simulink model "Drone_BBall_Developer"  (R2020a)
settings: Solver=FixedStepAuto  StartTime=0.0  StopTime=60  FixedStep=.001  RelTol=1e-3
values from neighbouring files (symbols this model uses):
  b = .25*m    (= 0.25)    [Run_Match.m]
  b_ball = .02*m_ball    (= 0.01)    [Run_Match.m]
  b_F_hook = 100    [Run_Match.m]
  b_F_hoop = m_ball * 50    (= 25)    [Run_Match.m]
  b_F_R = m * 20    (= 20)    [Run_Match.m]
  b_F_R_ball = m_ball * 10    (= 5)    [Run_Match.m]
  b_F_R_hook = m_hook * 100    (= 10)    [Run_Match.m]
  B_hook = r_hook^2*6*m_ball*g    (= 0.2943)    [Run_Match.m]
  b_hook = 0.05*m_hook    (= 0.005)    [Run_Match.m]
  b_tether = 1    [Run_Match.m]
  b_th = .1*J    (= 0.0192708333333)    [Run_Match.m]
  b_th_ball = .05*J_ball    (= 0.0009)    [Run_Match.m]
  b_x_net = 80*m_ball*g    (= 392.4)    [Run_Match.m]
  b_y_net = .4*m_ball*g    (= 1.962)    [Run_Match.m]
  drone = struct([])    [Run_Match.m]    (also in animate_drone_bball.m = [-r+w -r-w -r -r r r r+w r-w;             h    h  h  0 0 h  )
  g = 9.81    [Run_Match.m]
  J = 1/4*m*r^2 + 1/12*m*(2*(r+r_M_R))^2    (= 0.192708333333)    [Run_Match.m]
  J_ball = 2/5*m_ball*r_ball^2    (= 0.018)    [Run_Match.m]
  k_f = 4    [Run_Match.m]
  k_F_hook = 10000    [Run_Match.m]
  k_F_hoop = m_ball * 5000    (= 2500)    [Run_Match.m]
  k_F_R = m * 10000    (= 10000)    [Run_Match.m]
  k_F_R_ball = m_ball * 10000    (= 5000)    [Run_Match.m]
  k_F_R_hook = m_hook * 10000    (= 1000)    [Run_Match.m]
  k_tether = 40    [Run_Match.m]
  k_x_net = 200*m_ball*g    (= 981)    [Run_Match.m]
  k_y_net = .5*m_ball*g    (= 2.4525)    [Run_Match.m]
  L_tether = 1.0    (= 1)    [Run_Match.m]
  m = 1    [Run_Match.m]
  m_ball = .5    (= 0.5)    [Run_Match.m]
  m_hook = 0.1*m    (= 0.1)    [Run_Match.m]
  mu_f = .2    (= 0.2)    [Run_Match.m]
  mu_f_gnd = 0.5    [Run_Match.m]
  p_0 = [-5; 5]    [Run_Match.m]
  p_ball_0 = [0; r_ball]    [Run_Match.m]
  p_ball_dot_0 = [0; 12]    [Run_Match.m]
  p_emp = [0; -.4]    [Run_Match.m]
  p_emp_dot = [0; -5]    [Run_Match.m]
  p_hoop = [7.5 8; 8.5 8; -8.5 8; -7.5 8]'    [Run_Match.m]
  p_tether = [0; -0.259]    [Run_Match.m]
  r = 0.5    [Run_Match.m]    (also in animate_drone_bball.m = 0.475)
  r_ball = .3    (= 0.3)    [Run_Match.m]
  r_hook = 0.1    [Run_Match.m]
  r_M_R = 0.25*r    (= 0.125)    [Run_Match.m]
  T_0 = m*g    (= 9.81)    [Run_Match.m]
  T_max = 4*m*g    (= 39.24)    [Run_Match.m]
  T_tau = 0.1    [Run_Match.m]
undefined symbols (not defined in the file or in its folder): clock, M_max, sigbuilder_block, T_aux
libraries: dspswit3 x22, simulink x17, simulink_extras x3, dspmathops x2
(part 1 of 5)
settings Model: SimulationMode=accelerator  Creator=bsmith86  LastModifiedBy=Ivan
settings SolverCC: AlgebraicLoopSolver=LineSearch
settings DataIOCC: ReturnWorkspaceOutputs=off
settings DebuggingCC: ArithmeticOperatorsInVariantConditions=warning
settings SFSimCC: CustomCodeUndefinedFunction=UseInterfaceOnly
settings RTWCC: Description=Simulink Desktop Real-Time  SystemTargetFile=sldrt.tlc  TemplateMakefile=sldrt.tmf  RTWCompilerOptimization=on
settings CodeAppCC: MaxIdLength=95
settings TargetCC: TargetPreCompLibLocation=C:\Program Files\MATLAB\R2020a\toolbox\sldrt\lib\win64  TargetLangStandard=C99 (ISO)  SupportVariableSizeSignals=on

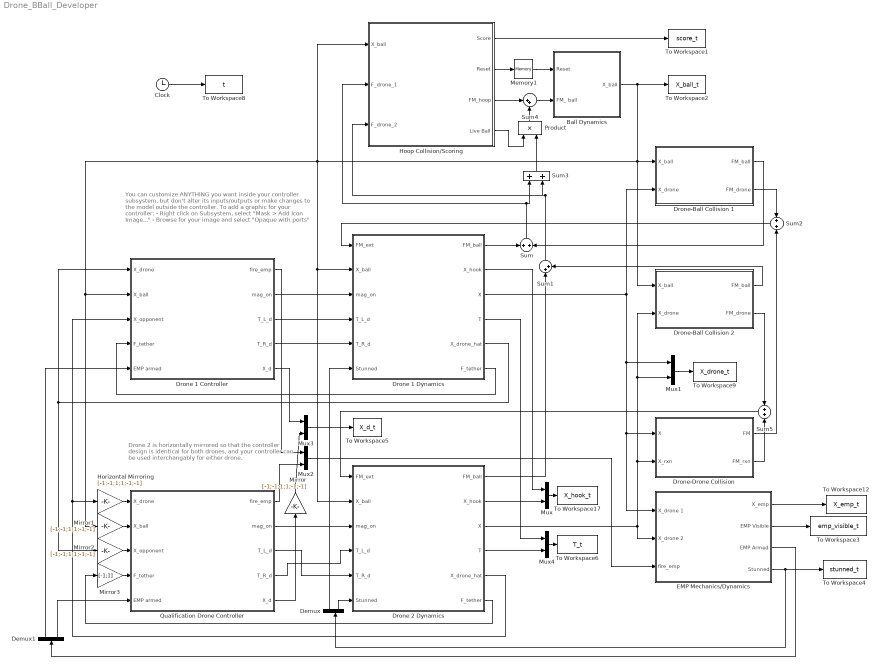
== system Drone_BBall_Developer ==
  note: Drone 2 is horizontally mirrored so that the controller design is identical for both drones, and your controller can be used interchangably for either drone.
  note: You can customize ANYTHING you want inside your controller subsystem, but don't alter its inputs/outputs or make changes to the model outside the controller.
      |
      | To add a graphic for your controller:
      | - Right click on Subsystem, select "Mask > Add Icon Image..."
      | - Browse for your image and select "Opaque with ports"
  " Mirror" : Gain  Gain=[-1;-1;1;1;-1;-1]
  Ball Dynamics : Subsystem
      mask Display: image('./graphics/ball_mask.png');
  Clock : Clock
  Demux : Demux  Outputs=2
  Demux1 : Demux  Outputs=2
  Drone 1 Controller : Subsystem
      mask Display: image('$imagefile'); % Use "Edit Image" on toolstrip to change.
  Drone 1 Dynamics : Subsystem  mask{param=drone(1)}
      mask prompts: param "Drone Parameter Structure"
      mask Display: image('./graphics/drone_mask_A.png');
  Drone 2 Dynamics : Subsystem  mask{param=drone(2)}
      mask prompts: param "Drone Parameter Structure"
      mask Display: image('./graphics/drone_mask_B.png');
  Drone-Ball Collision 1 : Subsystem  mask{r1=r_ball, r2=r, k_R=k_F_R, b_R=b_F_R}
      mask prompts: r1 "Radius of Object 1"; r2 "Radius of Object 2"; k_R "Collision Stiffness"; b_R "Collision Damping"
      mask Display: image('./graphics/collision_B_mask.png');
  Drone-Ball Collision 2 : Subsystem  mask{r1=r_ball, r2=r, k_R=k_F_R, b_R=b_F_R}
      mask prompts: r1 "Radius of Object 1"; r2 "Radius of Object 2"; k_R "Collision Stiffness"; b_R "Collision Damping"
      mask Display: image('./graphics/collision_B_mask.png');
  Drone-Drone Collision : Subsystem  mask{r1=r, r2=r, k_R=k_F_R, b_R=b_F_R}
      mask prompts: r1 "Radius of Object 1"; r2 "Radius of Object 2"; k_R "Collision Stiffness"; b_R "Collision Damping"
      mask Display: image('./graphics/collision_mask.png');
  EMP Mechanics/Dynamics : Subsystem
      mask Display: image('./graphics/emp_mask.png');
  Hoop Collision/Scoring : Subsystem
      mask Display: image('./graphics/backboard_mask.png'); % Use "Edit Image" on toolstrip to change.
  Horizontal Mirroring : Gain  Gain=[-1;-1;1;1;-1;-1]
  Memory1 : Memory
  Mirror1 : Gain  Gain=[-1;-1;1;1;-1;-1]
  Mirror2 : Gain  Gain=[-1;-1;1;1;-1;-1]
  Mirror3 : Gain  Gain=[-1;1]
  Mux{,1..4} (5 alike) : Mux  Inputs=2
  Product : Product
  Qualification Drone Controller : Subsystem
      mask help: Simulink:masks:GenSFuncDesc_MD
      mask Help: eval('feval(''rtwprivate'',''rtwhelpview'',''rtw_sfcn_block'')');
      mask Display: image('./graphics/ai_mask.png'); % Use "Edit Image" on toolstrip to change.
  Sum{,2..3,5} (4 alike) : Sum  Inputs=+|+
  Sum1 : Sum  Inputs=|++
  Sum4 : Sum  Inputs=|++
  To Workspace1 : ToWorkspace  VariableName=score_t  SampleTime=-1
  To Workspace12 : ToWorkspace  VariableName=X_emp_t  SampleTime=-1
  To Workspace17 : ToWorkspace  VariableName=X_hook_t  SampleTime=-1
  To Workspace2 : ToWorkspace  VariableName=X_ball_t  SampleTime=-1
  To Workspace3 : ToWorkspace  VariableName=emp_visible_t  SampleTime=-1
  To Workspace4 : ToWorkspace  VariableName=stunned_t  SampleTime=-1
  To Workspace5 : ToWorkspace  VariableName=X_d_t  SampleTime=-1
  To Workspace6 : ToWorkspace  VariableName=T_t  SampleTime=-1
  To Workspace8 : ToWorkspace  VariableName=t  SampleTime=-1
  To Workspace9 : ToWorkspace  VariableName=X_drone_t  SampleTime=-1
  wires:
  Sum4/1 -> Ball Dynamics/2(FM_ ball)
  Hoop Collision/Scoring/3(FM_hoop) -> Sum4/1
  Hoop Collision/Scoring/2(Reset) -> Memory1/1
  Hoop Collision/Scoring/1(Score) -> To Workspace1/1
  Hoop Collision/Scoring/4(Live Ball) -> Product/1
  Product/1 -> Sum4/2
  Ball Dynamics/1(" X_ball") -> To Workspace2/1, Drone-Ball Collision 1/1(X_ball), Drone-Ball Collision 2/1(X_ball), Hoop Collision/Scoring/1(X_ball), Drone 1 Dynamics/2(X_ball), Drone 2 Dynamics/2(X_ball), Drone 1 Controller/2(X_ball), Mirror1/1
  Memory1/1 -> Ball Dynamics/1(Reset)
  EMP Mechanics/Dynamics/4(Stunned) -> Demux/1, To Workspace4/1
  Demux/2 -> Drone 2 Dynamics/6(Stunned)
  Drone 1 Controller/2(mag_on) -> Drone 1 Dynamics/3(mag_on)
  Demux/1 -> Drone 1 Dynamics/6(Stunned)
  Drone 1 Controller/3(T_L_d) -> Drone 1 Dynamics/4(T_L_d)
  Drone 1 Controller/4(T_R_d) -> Drone 1 Dynamics/5(T_R_d)
  Drone 1 Dynamics/5(X_drone_hat) -> Drone 1 Controller/1(X_drone), Mirror2/1
  Drone 1 Dynamics/3(X) -> Drone-Ball Collision 1/2(X_drone), EMP Mechanics/Dynamics/1(X_drone 1), Drone-Drone Collision/1(X), Mux1/1
  Qualification Drone Controller/4(T_R_d) -> Drone 2 Dynamics/4(T_L_d)
  Qualification Drone Controller/3(T_L_d) -> Drone 2 Dynamics/5(T_R_d)
  Qualification Drone Controller/2(mag_on) -> Drone 2 Dynamics/3(mag_on)
  Drone 1 Dynamics/1(FM_ball) -> Sum/1
  Mux/1 -> To Workspace17/1
  Mux1/1 -> To Workspace9/1
  Drone 1 Dynamics/2(X_hook) -> Mux/1
  Drone 2 Dynamics/2(X_hook) -> Mux/2
  Drone 2 Dynamics/3(X) -> EMP Mechanics/Dynamics/2(X_drone 2), Drone-Ball Collision 2/2(X_drone), Mux1/2, Drone-Drone Collision/2(X_rxn)
  EMP Mechanics/Dynamics/1(X_emp) -> To Workspace12/1
  EMP Mechanics/Dynamics/2(EMP Visible) -> To Workspace3/1
  Drone-Ball Collision 2/1(FM_ball) -> Sum1/2
  Drone-Ball Collision 1/1(FM_ball) -> Sum/2
  Drone-Ball Collision 1/2(FM_drone) -> Sum2/1
  Drone-Drone Collision/1(FM) -> Sum2/2
  Drone-Drone Collision/2(FM_rxn) -> Sum5/2
  Drone-Ball Collision 2/2(FM_drone) -> Sum5/1
  Sum2/1 -> Drone 1 Dynamics/1(FM_ext)
  Sum5/1 -> Drone 2 Dynamics/1(FM_ext)
  Clock/1 -> To Workspace8/1
  EMP Mechanics/Dynamics/3(EMP Armed) -> Demux1/1
  Drone 2 Dynamics/5(X_drone_hat) -> Drone 1 Controller/3(X_opponent), Horizontal Mirroring/1
  Horizontal Mirroring/1 -> Qualification Drone Controller/1(X_drone)
  Mirror1/1 -> Qualification Drone Controller/2(X_ball)
  Mirror2/1 -> Qualification Drone Controller/3(X_opponent)
  Demux1/2 -> Qualification Drone Controller/5(EMP armed)
  Demux1/1 -> Drone 1 Controller/5(EMP armed)
  Drone 1 Dynamics/6(F_tether) -> Drone 1 Controller/4(F_tether)
  Drone 2 Dynamics/6(F_tether) -> Mirror3/1
  Mirror3/1 -> Qualification Drone Controller/4(F_tether)
  Mux2/1 -> EMP Mechanics/Dynamics/3(fire_emp)
  Drone 1 Controller/1(fire_emp) -> Mux2/1
  Qualification Drone Controller/1(fire_emp) -> Mux2/2
  Drone 1 Controller/5(X_d) -> Mux3/1
  Qualification Drone Controller/5(X_d) -> " Mirror"/1
  Mux3/1 -> To Workspace5/1
  " Mirror"/1 -> Mux3/2
  Mux4/1 -> To Workspace6/1
  Drone 2 Dynamics/4(T) -> Mux4/2
  Drone 1 Dynamics/4(T) -> Mux4/1
  Drone 2 Dynamics/1(FM_ball) -> Sum1/1
  Sum1/1 -> Hoop Collision/Scoring/3(F_drone_2), Sum3/2
  Sum/1 -> Hoop Collision/Scoring/2(F_drone_1), Sum3/1
  Sum3/1 -> Product/2

== system Drone_BBall_Developer/Ball Dynamics ==
  Reset : Inport
  FM_ ball : Inport  Port=2
  Band-Limited White Noise : simulink/Sources/Band-Limited White Noise  Cov=[0.001^2]  Ts=0.1  seed=round(sum(clock))
  Band-Limited White Noise1 : simulink/Sources/Band-Limited White Noise  Cov=[0.001^2]  Ts=0.1  seed=round(sum(clock))+1
  Band-Limited White Noise2 : simulink/Sources/Band-Limited White Noise  Cov=[(.001*r_ball)^2]  Ts=0.1  seed=round(sum(clock))+2
  Ceiling Reactions : Subsystem
  Constant : Constant  Value=[0;-m_ball*g]
  Demux : Demux  Outputs=3
  Demux1 : Demux  Outputs=2
  Demux2 : Demux  Outputs=2
  Ground Reactions : Subsystem
  Left Wall Reactions : Subsystem
  Linear Dynamics : Subsystem
  Mux : Mux  Inputs=2
  Mux1 : Mux  Inputs=6
  Mux2 : Mux  Inputs=3
  Right Wall Reactions : Subsystem
  Rotational Dynamics : Subsystem
  Scope : Scope
  Sum : Sum  Inputs=+|+
  Sum1 : Sum  Inputs=+|+||+||+||+
  Sum2 : Sum  Inputs=|++
  " X_ball" : Outport  VectorParamsAs1DForOutWhenUnconnected=off
  wires:
  Rotational Dynamics/2(theta_dot) -> Mux1/6  "theta_dot"
  Rotational Dynamics/1(theta) -> Mux1/5  "theta"
  Mux1/1 -> " X_ball"/1, Ceiling Reactions/1(X), Ground Reactions/1(X), Left Wall Reactions/1(X), Right Wall Reactions/1(X)
  Sum/1 -> Linear Dynamics/2(F)
  Constant/1 -> Sum/1
  Linear Dynamics/1(p) -> Demux1/1  "p"
  Linear Dynamics/2(p_dot) -> Demux2/1  "p_dot"
  Demux1/1 -> Mux1/1  "x"
  Demux1/2 -> Mux1/3  "y"
  Demux2/1 -> Mux1/2  "x_dot"
  Demux2/2 -> Mux1/4  "y_dot"
  Reset/1 -> Rotational Dynamics/1(Reset), Linear Dynamics/1(Reset)
  FM_ ball/1 -> Sum1/1
  Demux/1 -> Mux/1
  Demux/2 -> Mux/2
  Mux/1 -> Sum/2
  Demux/3 -> Rotational Dynamics/2(M)
  Sum1/1 -> Sum2/1
  Ground Reactions/1(FM_R) -> Sum1/2
  Left Wall Reactions/1(FM_R) -> Sum1/3
  Right Wall Reactions/1(FM_R) -> Sum1/4
  Ceiling Reactions/1(FM_R) -> Sum1/5
  Band-Limited White Noise2/1 -> Mux2/3
  Band-Limited White Noise1/1 -> Mux2/2
  Band-Limited White Noise/1 -> Mux2/1
  Sum2/1 -> Demux/1
  Mux2/1 -> Sum2/2, Scope/1

== system Drone_BBall_Developer/Drone 1 Controller ==
  X_drone : Inport
  X_ball : Inport  Port=2
  X_opponent : Inport  Port=3
  F_tether : Inport  Port=4
  EMP armed : Inport  Port=5
  Clock : Clock
  Clock1 : Clock
  Detect Ball in Freefall : Subsystem  mask(Detect Object in Freefall){g_tol=4}
      mask prompts: g_tol "Tolerance for g (m/s^2)"
      mask help:
      | Estimates the vertical acceleration of an object to determine when it is in freefall.
      | Judges the object to be in freefall if its vertical acceleration is within a given tolerance of 9.81 m/s^2.
  EMP Controller : MATLAB Function  TreatAsAtomicUnit=on
  Finite State Machine : MATLAB Function  TreatAsAtomicUnit=on
  Flipover Decector : MATLAB Function  TreatAsAtomicUnit=on
  Magnet Controller : MATLAB Function  TreatAsAtomicUnit=on
  Manual Switch : ManualSwitch
  Manual Switch1 : ManualSwitch
  Manual Switch2 : ManualSwitch
  Memory{,1,3..4} (4 alike) : Memory
  Memory2 : Memory  InitialCondition=1
  Mux : Mux  Inputs=6
  Posession Detection : MATLAB Function  TreatAsAtomicUnit=on
  Preamp to smooth p_d(t) (Double click to tune) : Subsystem  mask{zeta_x=0.7, zeta_y=0.7, zeta_th=0.7, omega_x=1, omega_y=2, omega_th=20}
      mask prompts: zeta_x "damping ratio for x_d(t)"; zeta_y "damping ratio for y_d(t)"; zeta_th "damping ratio for theta_d(t)"; omega_x "natrual frequency for x_d(t)"; omega_y "natrual frequency for y_d(t)"; omega_th "natrual frequency for theta_d(t)"
      mask DialogControl DescGroupVar Prompt: Preamp to Smooth Reference Input
      mask DialogControl Instructions Prompt: This preamp filter smooths the raw values of the reference input signals x_d(t) and y_d(t), resulting in an easier reference trajectory for the drone dynamical controller to follow. This allows for abrupt changes in the raw signals for x_d(t) and y_d(t). Tune the damping ratio (zeta) and undamped natural frequency (omega_n) of the preamp for each dimension of the reference input to set the agressiveness of the cotnroller.
  Predict Catch Position : MATLAB Function  TreatAsAtomicUnit=on
  Quadcopter Dynamical Controller : Subsystem
  Quadcopter Dynamical Controller (Arena Frame) : Subsystem  Commented=on
  Quadcopter Dynamical Controller (Drone Frame) : Subsystem  Commented=on
  Reference Inputs for Testing : Subsystem  Tag=STV Subsys  LoadFcn=sigbuilder_block('load');  StartFcn=sigbuilder_block('start');  StopFcn=sigbuilder_block('stop');  ClipboardFcn=sigbuilder_block('clipboard');  mask(Sigbuilder block){tuvar=[0:10]}
      mask help: Simulink:masks:SigbuilderBlock_MD
      mask init:
      | if ~strcmp(get_param(bdroot(gcbh),'SimulationStatus'),'stopped') tuvar = sigbuilder_block('maskInit'); end
      settings: CopyFcn=sigbuilder_block('copy');  DeleteFcn=sigbuilder_block('delete');  ModelCloseFcn=sigbuilder_block('modelClose');  PreSaveFcn=sigbuilder_block('preSave');  PauseFcn=sigbuilder_block('pause');  ContinueFcn=sigbuilder_block('continue');  NameChangeFcn=sigbuilder_block('namechange');  OpenFcn=sigbuilder_block('open',[-8.25 87 476.625 499.125 ]);  CloseFcn=sigbuilder_block('close');
      mask Display: plot(0, 0, 100, 100,[2, 2, 32, 32, 2], [68, 8, 8, 68, 68],[32, 2], [38, 38], [32, 19, 2],[53, 60, 44], [32, 17, 17, 2],[16, 16, 31, 31]);txt = getActiveGroup(gcbh);text(2, 100, txt,'verticalAlignment', 'top');
  Sum : Sum  Inputs=|++
  Switch : Switch  Criteria=u2 ~= 0
  Useful Scopes for Troubleshooting : Subsystem
  Zero : Constant  Value=0  OutDataTypeStr=Inherit: Inherit via back propagation
  Zero1 : Constant  Value=0  OutDataTypeStr=Inherit: Inherit via back propagation
  t_catch : Scope
  fire_emp : Outport  VectorParamsAs1DForOutWhenUnconnected=off
  mag_on : Outport  Port=2  VectorParamsAs1DForOutWhenUnconnected=off
  T_L_d : Outport  Port=3  VectorParamsAs1DForOutWhenUnconnected=off
  T_R_d : Outport  Port=4  VectorParamsAs1DForOutWhenUnconnected=off
  X_d : Outport  Port=5  VectorParamsAs1DForOutWhenUnconnected=off
  wires:
  Magnet Controller/1(mag_on) -> Manual Switch2/1
  Clock/1 -> Magnet Controller/2(t)
  Memory/1 -> Magnet Controller/3(t_hold_prev)
  Magnet Controller/2(t_hold) -> Memory/1
  X_drone/1 -> Quadcopter Dynamical Controller/1(X), Flipover Decector/1(X_drone), Useful Scopes for Troubleshooting/1(X), Finite State Machine/1(X_drone), EMP Controller/1(X_drone), Predict Catch Position/1(X_drone), Posession Detection/1(X_drone)
  Reference Inputs for Testing/4(fire_emp) -> Manual Switch1/2
  Reference Inputs for Testing/5(mag_on) -> Manual Switch2/2
  EMP armed/1 -> EMP Controller/3(emp_armed)
  F_tether/1 -> Posession Detection/3(F_tether)
  Finite State Machine/1(X_d) -> Manual Switch/1
  Manual Switch1/1 -> fire_emp/1
  Manual Switch2/1 -> Finite State Machine/6(mag_on), mag_on/1
  Posession Detection/1(possession) -> Memory1/1, Finite State Machine/3(possession)
  Memory1/1 -> Posession Detection/4(possession_prev)
  Finite State Machine/2(state) -> Memory2/1
  Memory2/1 -> Finite State Machine/7(state_prev)
  X_ball/1 -> Magnet Controller/1(X_ball), Detect Ball in Freefall/1(X), Predict Catch Position/2(X_ball), Posession Detection/2(X_ball), Finite State Machine/2(X_ball)
  X_opponent/1 -> EMP Controller/2(X_opponent)
  EMP Controller/1(fire_emp) -> Manual Switch1/1
  Flipover Decector/1(flip) -> Memory3/1, Switch/2  "Disable right rotor to flip"
  Memory3/1 -> Flipover Decector/2(flip_prev)
  Zero/1 -> Switch/1
  Quadcopter Dynamical Controller/2(T_R_d) -> Switch/3
  Quadcopter Dynamical Controller/3(X_d_adj) -> Useful Scopes for Troubleshooting/2(X_d), X_d/1
  Quadcopter Dynamical Controller/1(T_L_d) -> T_L_d/1
  Switch/1 -> T_R_d/1
  Reference Inputs for Testing/1(x_d) -> Mux/1
  Reference Inputs for Testing/2(y_d) -> Mux/3
  Mux/1 -> Manual Switch/2
  Reference Inputs for Testing/3(theta_d) -> Mux/5
  Preamp to smooth p_d(t) (Double click to tune)/1(X_d(t)) -> Quadcopter Dynamical Controller/2(X_d)
  Detect Ball in Freefall/1(Object in Freefall) -> Finite State Machine/5(freefall)
  Memory4/1 -> Predict Catch Position/3(t_catch_prev)
  Predict Catch Position/1(X_catch) -> Finite State Machine/4(X_catch)
  Predict Catch Position/2(t_catch) -> Sum/1, Memory4/1
  Sum/1 -> t_catch/1
  Clock1/1 -> Sum/2
  Manual Switch/1 -> Preamp to smooth p_d(t) (Double click to tune)/1(X_d_raw(t))
  Zero1/1 -> Mux/6, Mux/4, Mux/2

== system Drone_BBall_Developer/Drone 1 Dynamics ==
  FM_ext : Inport
  X_ball : Inport  Port=2
  mag_on : Inport  Port=3
  T_L_d : Inport  Port=4
  T_R_d : Inport  Port=5
  Stunned : Inport  Port=6
  AND : Logic  AllPortsSameDT=off  OutDataTypeStr=boolean
  Constant : Constant  Value=0.001
  Constant1 : Constant  Value=0.1
  Hook Plant : Subsystem
  NOT : Logic  Operator=NOT  IconShape=distinctive  AllPortsSameDT=off  OutDataTypeStr=boolean
  Quadcopter Plant : Subsystem
  Sum : Sum  Inputs=++|
  Switch : Switch  Criteria=u2 ~= 0
  Variable Time Delay : VariableTransportDelay  MaximumDelay=10  InitialOutput=param.X_0  MaximumPoints=10240  ZeroDelay=on  TransDelayFeedthrough=on
  FM_ball : Outport  VectorParamsAs1DForOutWhenUnconnected=off
  X_hook : Outport  Port=2  VectorParamsAs1DForOutWhenUnconnected=off
  X : Outport  Port=3  VectorParamsAs1DForOutWhenUnconnected=off
  T : Outport  Port=4  VectorParamsAs1DForOutWhenUnconnected=off
  X_drone_hat : Outport  Port=5  VectorParamsAs1DForOutWhenUnconnected=off
  F_tether : Outport  Port=6  VectorParamsAs1DForOutWhenUnconnected=off
  wires:
  T_L_d/1 -> Quadcopter Plant/2(T_L_d)
  Hook Plant/2(FM_ball) -> FM_ball/1
  Constant1/1 -> Switch/1
  Constant/1 -> Switch/3
  Switch/1 -> Variable Time Delay/2
  Variable Time Delay/1 -> X_drone_hat/1
  X_ball/1 -> Hook Plant/2(X_ball)
  Stunned/1 -> Switch/2, NOT/1
  T_R_d/1 -> Quadcopter Plant/3(T_R_d)
  Hook Plant/1(X_hook) -> X_hook/1
  Sum/1 -> Quadcopter Plant/1(FM_ext)
  FM_ext/1 -> Sum/2
  Quadcopter Plant/1(X_drone) -> X/1, Hook Plant/3(X_drone), Variable Time Delay/1
  NOT/1 -> AND/1
  AND/1 -> Hook Plant/1(mag_on)
  mag_on/1 -> AND/2
  Hook Plant/4(FM_tether_rxn) -> Sum/1
  Hook Plant/3(F_tether_r) -> F_tether/1
  Quadcopter Plant/2(T) -> T/1

== system Drone_BBall_Developer/Drone 2 Dynamics ==
  FM_ext : Inport
  X_ball : Inport  Port=2
  mag_on : Inport  Port=3
  T_L_d : Inport  Port=4
  T_R_d : Inport  Port=5
  Stunned : Inport  Port=6
  AND : Logic  AllPortsSameDT=off  OutDataTypeStr=boolean
  Constant : Constant  Value=0.001
  Constant1 : Constant  Value=0.1
  Gain : Gain  Gain=-1
  Hook Plant : Subsystem
  NOT : Logic  Operator=NOT  IconShape=distinctive  AllPortsSameDT=off  OutDataTypeStr=boolean
  Quadcopter Plant : Subsystem
  Sum : Sum  Inputs=++|
  Switch : Switch  Criteria=u2 ~= 0
  Variable Time Delay : VariableTransportDelay  MaximumDelay=10  InitialOutput=param.X_0  MaximumPoints=10240  ZeroDelay=on  TransDelayFeedthrough=on
  FM_ball : Outport  VectorParamsAs1DForOutWhenUnconnected=off
  X_hook : Outport  Port=2  VectorParamsAs1DForOutWhenUnconnected=off
  X : Outport  Port=3  VectorParamsAs1DForOutWhenUnconnected=off
  T : Outport  Port=4  VectorParamsAs1DForOutWhenUnconnected=off
  X_drone_hat : Outport  Port=5  VectorParamsAs1DForOutWhenUnconnected=off
  F_tether : Outport  Port=6  VectorParamsAs1DForOutWhenUnconnected=off
  wires:
  T_L_d/1 -> Quadcopter Plant/2(T_L_d)
  Hook Plant/2(FM_ball) -> FM_ball/1
  Constant1/1 -> Switch/1
  Hook Plant/4(FM_tether) -> Gain/1
  Constant/1 -> Switch/3
  Switch/1 -> Variable Time Delay/2
  Variable Time Delay/1 -> X_drone_hat/1
  X_ball/1 -> Hook Plant/2(X_ball)
  Stunned/1 -> Switch/2, NOT/1
  T_R_d/1 -> Quadcopter Plant/3(T_R_d)
  Hook Plant/1(X_hook) -> X_hook/1
  Sum/1 -> Quadcopter Plant/1(FM_ext)
  FM_ext/1 -> Sum/2
  Quadcopter Plant/1(X_drone) -> X/1, Hook Plant/3(X_drone), Variable Time Delay/1
  NOT/1 -> AND/1
  AND/1 -> Hook Plant/1(mag_on)
  mag_on/1 -> AND/2
  Gain/1 -> Sum/1
  Hook Plant/3(F_tether_r) -> F_tether/1
  Quadcopter Plant/2(T) -> T/1

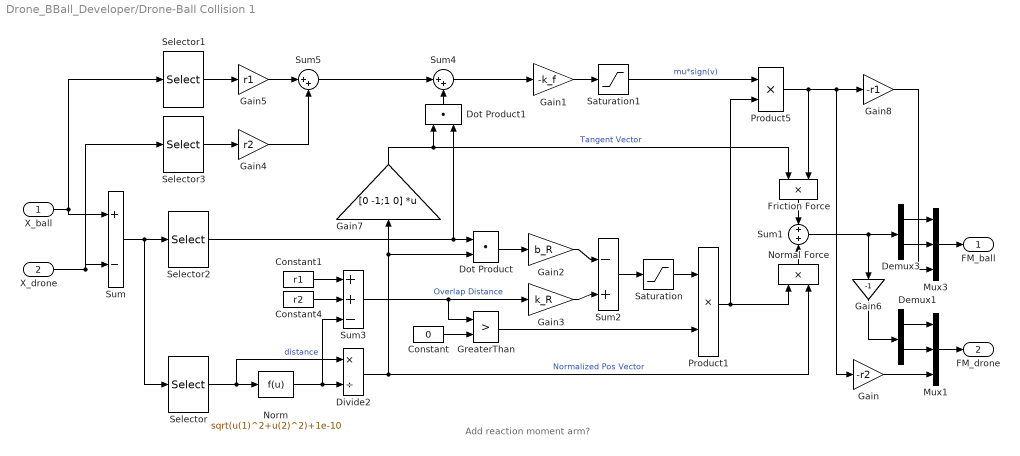
== system Drone_BBall_Developer/Drone-Ball Collision 1 ==
  note: Add reaction moment arm?
  X_ball : Inport
  X_drone : Inport  Port=2
  Constant : Constant  Value=0
  Constant1 : Constant  Value=r1
  Constant4 : Constant  Value=r2
  Demux1 : Demux  Outputs=2
  Demux3 : Demux  Outputs=2
  Divide2 : Product  Inputs=*/
  Dot Product : DotProduct  InputSameDT=on  OutDataTypeStr=Inherit: Inherit via internal rule
  Dot Product1 : DotProduct  InputSameDT=on  OutDataTypeStr=Inherit: Inherit via internal rule
  Friction Force : Product
  Gain : Gain  Gain=-r2
  Gain1 : Gain  Gain=-k_f
  Gain2 : Gain  Gain=b_R
  Gain3 : Gain  Gain=k_R
  Gain4 : Gain  Gain=r2
  Gain5 : Gain  Gain=r1
  Gain6 : Gain  Gain=-1
  Gain7 : Gain  Gain=[0 -1;1 0]  Multiplication=Matrix(K*u)
  Gain8 : Gain  Gain=-r1
  GreaterThan : RelationalOperator  Operator=>  OutDataTypeStr=boolean  RndMeth=Simplest
  Mux1 : Mux  Inputs=3
  Mux3 : Mux  Inputs=3
  Norm : Fcn  Expr=sqrt(u(1)^2+u(2)^2)+1e-10
  Normal Force : Product
  Product1 : Product
  Product5 : Product
  Saturation : Saturate  UpperLimit=Inf  LowerLimit=0
  Saturation1 : Saturate  UpperLimit=mu_f  LowerLimit=-mu_f
  Selector : Selector  InputPortWidth=6  IndexOptions=Index vector (dialog)  Indices=[1 3]  OutputSizes=1
  Selector1 : Selector  InputPortWidth=6  IndexOptions=Index vector (dialog)  Indices=[6]  OutputSizes=1
  Selector2 : Selector  InputPortWidth=6  IndexOptions=Index vector (dialog)  Indices=[2 4]  OutputSizes=1
  Selector3 : Selector  InputPortWidth=6  IndexOptions=Index vector (dialog)  Indices=[6]  OutputSizes=1
  Sum : Sum  Inputs=+|-
  Sum1 : Sum  Inputs=+|+
  Sum2 : Sum  Inputs=-|+
  Sum3 : Sum  Inputs=++-
  Sum4 : Sum  Inputs=|++
  Sum5 : Sum  Inputs=|++
  FM_ball : Outport  VectorParamsAs1DForOutWhenUnconnected=off
  FM_drone : Outport  Port=2  VectorParamsAs1DForOutWhenUnconnected=off
  wires:
  Gain8/1 -> Mux3/3
  X_ball/1 -> Sum/1, Selector1/1
  X_drone/1 -> Selector3/1, Sum/2
  Sum/1 -> Selector/1, Selector2/1
  Selector/1 -> Norm/1, Divide2/1
  Sum3/1 -> GreaterThan/1, Gain3/1  "Overlap Distance"
  Constant/1 -> GreaterThan/2
  GreaterThan/1 -> Product1/2
  Dot Product/1 -> Gain2/1
  Gain2/1 -> Sum2/1
  Gain3/1 -> Sum2/2
  Product5/1 -> Gain/1, Gain8/1, Friction Force/2
  Norm/1 -> Sum3/3, Divide2/2  "distance"
  Constant4/1 -> Sum3/2
  Divide2/1 -> Normal Force/2, Gain7/1, Dot Product/2  "Normalized Pos Vector"
  Gain7/1 -> Friction Force/1, Dot Product1/1  "Tangent Vector"
  Selector1/1 -> Gain5/1
  Gain1/1 -> Saturation1/1
  Normal Force/1 -> Sum1/2
  Friction Force/1 -> Sum1/1
  Product1/1 -> Normal Force/1, Product5/2
  Sum2/1 -> Saturation/1
  Saturation1/1 -> Product5/1  "mu*sign(v)"
  Demux3/1 -> Mux3/1
  Demux3/2 -> Mux3/2
  Selector3/1 -> Gain4/1
  Gain5/1 -> Sum5/1
  Gain4/1 -> Sum5/2
  Sum1/1 -> Demux3/1, Gain6/1
  Demux1/1 -> Mux1/1
  Demux1/2 -> Mux1/2
  Gain/1 -> Mux1/3
  Gain6/1 -> Demux1/1
  Constant1/1 -> Sum3/1
  Sum5/1 -> Sum4/1
  Selector2/1 -> Dot Product/1, Dot Product1/2
  Sum4/1 -> Gain1/1
  Mux3/1 -> FM_ball/1
  Mux1/1 -> FM_drone/1
  Saturation/1 -> Product1/1
  Dot Product1/1 -> Sum4/2

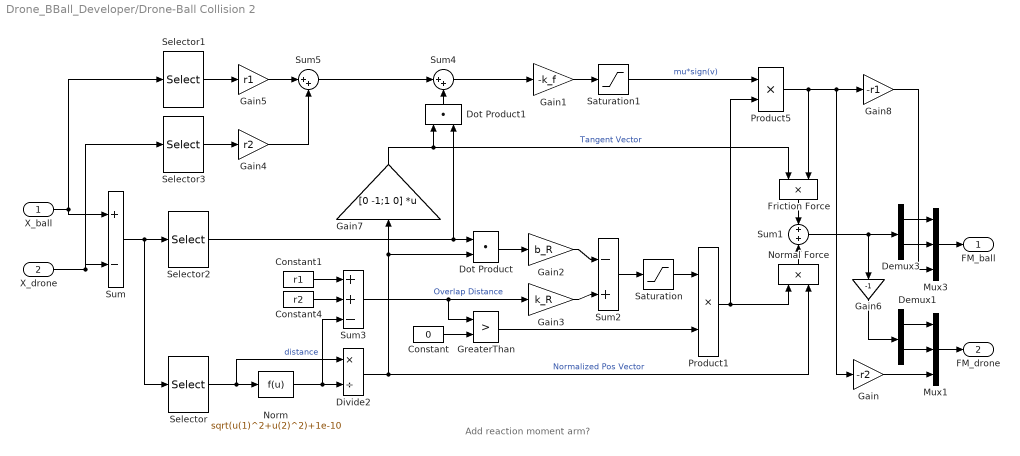
== system Drone_BBall_Developer/Drone-Ball Collision 2 ==
  note: Add reaction moment arm?
  X_ball : Inport
  X_drone : Inport  Port=2
  Constant : Constant  Value=0
  Constant1 : Constant  Value=r1
  Constant4 : Constant  Value=r2
  Demux1 : Demux  Outputs=2
  Demux3 : Demux  Outputs=2
  Divide2 : Product  Inputs=*/
  Dot Product : DotProduct  InputSameDT=on  OutDataTypeStr=Inherit: Inherit via internal rule
  Dot Product1 : DotProduct  InputSameDT=on  OutDataTypeStr=Inherit: Inherit via internal rule
  Friction Force : Product
  Gain : Gain  Gain=-r2
  Gain1 : Gain  Gain=-k_f
  Gain2 : Gain  Gain=b_R
  Gain3 : Gain  Gain=k_R
  Gain4 : Gain  Gain=r2
  Gain5 : Gain  Gain=r1
  Gain6 : Gain  Gain=-1
  Gain7 : Gain  Gain=[0 -1;1 0]  Multiplication=Matrix(K*u)
  Gain8 : Gain  Gain=-r1
  GreaterThan : RelationalOperator  Operator=>  OutDataTypeStr=boolean  RndMeth=Simplest
  Mux1 : Mux  Inputs=3
  Mux3 : Mux  Inputs=3
  Norm : Fcn  Expr=sqrt(u(1)^2+u(2)^2)+1e-10
  Normal Force : Product
  Product1 : Product
  Product5 : Product
  Saturation : Saturate  UpperLimit=Inf  LowerLimit=0
  Saturation1 : Saturate  UpperLimit=mu_f  LowerLimit=-mu_f
  Selector : Selector  InputPortWidth=6  IndexOptions=Index vector (dialog)  Indices=[1 3]  OutputSizes=1
  Selector1 : Selector  InputPortWidth=6  IndexOptions=Index vector (dialog)  Indices=[6]  OutputSizes=1
  Selector2 : Selector  InputPortWidth=6  IndexOptions=Index vector (dialog)  Indices=[2 4]  OutputSizes=1
  Selector3 : Selector  InputPortWidth=6  IndexOptions=Index vector (dialog)  Indices=[6]  OutputSizes=1
  Sum : Sum  Inputs=+|-
  Sum1 : Sum  Inputs=+|+
  Sum2 : Sum  Inputs=-|+
  Sum3 : Sum  Inputs=++-
  Sum4 : Sum  Inputs=|++
  Sum5 : Sum  Inputs=|++
  FM_ball : Outport  VectorParamsAs1DForOutWhenUnconnected=off
  FM_drone : Outport  Port=2  VectorParamsAs1DForOutWhenUnconnected=off
  wires:
  Gain8/1 -> Mux3/3
  X_ball/1 -> Sum/1, Selector1/1
  X_drone/1 -> Selector3/1, Sum/2
  Sum/1 -> Selector/1, Selector2/1
  Selector/1 -> Norm/1, Divide2/1
  Sum3/1 -> GreaterThan/1, Gain3/1  "Overlap Distance"
  Constant/1 -> GreaterThan/2
  GreaterThan/1 -> Product1/2
  Dot Product/1 -> Gain2/1
  Gain2/1 -> Sum2/1
  Gain3/1 -> Sum2/2
  Product5/1 -> Gain/1, Gain8/1, Friction Force/2
  Norm/1 -> Sum3/3, Divide2/2  "distance"
  Constant4/1 -> Sum3/2
  Divide2/1 -> Normal Force/2, Gain7/1, Dot Product/2  "Normalized Pos Vector"
  Gain7/1 -> Friction Force/1, Dot Product1/1  "Tangent Vector"
  Selector1/1 -> Gain5/1
  Gain1/1 -> Saturation1/1
  Normal Force/1 -> Sum1/2
  Friction Force/1 -> Sum1/1
  Product1/1 -> Normal Force/1, Product5/2
  Sum2/1 -> Saturation/1
  Saturation1/1 -> Product5/1  "mu*sign(v)"
  Demux3/1 -> Mux3/1
  Demux3/2 -> Mux3/2
  Selector3/1 -> Gain4/1
  Gain5/1 -> Sum5/1
  Gain4/1 -> Sum5/2
  Sum1/1 -> Demux3/1, Gain6/1
  Demux1/1 -> Mux1/1
  Demux1/2 -> Mux1/2
  Gain/1 -> Mux1/3
  Gain6/1 -> Demux1/1
  Constant1/1 -> Sum3/1
  Sum5/1 -> Sum4/1
  Selector2/1 -> Dot Product/1, Dot Product1/2
  Sum4/1 -> Gain1/1
  Mux3/1 -> FM_ball/1
  Mux1/1 -> FM_drone/1
  Saturation/1 -> Product1/1
  Dot Product1/1 -> Sum4/2

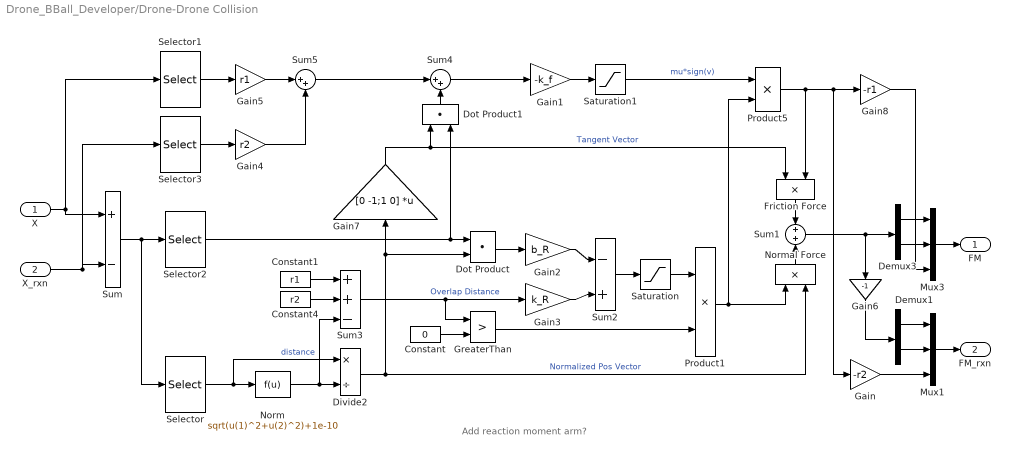
== system Drone_BBall_Developer/Drone-Drone Collision ==
  note: Add reaction moment arm?
  X : Inport
  X_rxn : Inport  Port=2
  Constant : Constant  Value=0
  Constant1 : Constant  Value=r1
  Constant4 : Constant  Value=r2
  Demux1 : Demux  Outputs=2
  Demux3 : Demux  Outputs=2
  Divide2 : Product  Inputs=*/
  Dot Product : DotProduct  InputSameDT=on  OutDataTypeStr=Inherit: Inherit via internal rule
  Dot Product1 : DotProduct  InputSameDT=on  OutDataTypeStr=Inherit: Inherit via internal rule
  Friction Force : Product
  Gain : Gain  Gain=-r2
  Gain1 : Gain  Gain=-k_f
  Gain2 : Gain  Gain=b_R
  Gain3 : Gain  Gain=k_R
  Gain4 : Gain  Gain=r2
  Gain5 : Gain  Gain=r1
  Gain6 : Gain  Gain=-1
  Gain7 : Gain  Gain=[0 -1;1 0]  Multiplication=Matrix(K*u)
  Gain8 : Gain  Gain=-r1
  GreaterThan : RelationalOperator  Operator=>  OutDataTypeStr=boolean  RndMeth=Simplest
  Mux1 : Mux  Inputs=3
  Mux3 : Mux  Inputs=3
  Norm : Fcn  Expr=sqrt(u(1)^2+u(2)^2)+1e-10
  Normal Force : Product
  Product1 : Product
  Product5 : Product
  Saturation : Saturate  UpperLimit=Inf  LowerLimit=0
  Saturation1 : Saturate  UpperLimit=mu_f  LowerLimit=-mu_f
  Selector : Selector  InputPortWidth=6  IndexOptions=Index vector (dialog)  Indices=[1 3]  OutputSizes=1
  Selector1 : Selector  InputPortWidth=6  IndexOptions=Index vector (dialog)  Indices=[6]  OutputSizes=1
  Selector2 : Selector  InputPortWidth=6  IndexOptions=Index vector (dialog)  Indices=[2 4]  OutputSizes=1
  Selector3 : Selector  InputPortWidth=6  IndexOptions=Index vector (dialog)  Indices=[6]  OutputSizes=1
  Sum : Sum  Inputs=+|-
  Sum1 : Sum  Inputs=+|+
  Sum2 : Sum  Inputs=-|+
  Sum3 : Sum  Inputs=++-
  Sum4 : Sum  Inputs=|++
  Sum5 : Sum  Inputs=|++
  FM : Outport  VectorParamsAs1DForOutWhenUnconnected=off
  FM_rxn : Outport  Port=2  VectorParamsAs1DForOutWhenUnconnected=off
  wires:
  Gain8/1 -> Mux3/3
  X/1 -> Sum/1, Selector1/1
  X_rxn/1 -> Selector3/1, Sum/2
  Sum/1 -> Selector/1, Selector2/1
  Selector/1 -> Norm/1, Divide2/1
  Sum3/1 -> GreaterThan/1, Gain3/1  "Overlap Distance"
  Constant/1 -> GreaterThan/2
  GreaterThan/1 -> Product1/2
  Dot Product/1 -> Gain2/1
  Gain2/1 -> Sum2/1
  Gain3/1 -> Sum2/2
  Product5/1 -> Gain/1, Gain8/1, Friction Force/2
  Norm/1 -> Sum3/3, Divide2/2  "distance"
  Constant4/1 -> Sum3/2
  Divide2/1 -> Normal Force/2, Gain7/1, Dot Product/2  "Normalized Pos Vector"
  Gain7/1 -> Friction Force/1, Dot Product1/1  "Tangent Vector"
  Selector1/1 -> Gain5/1
  Gain1/1 -> Saturation1/1
  Normal Force/1 -> Sum1/2
  Friction Force/1 -> Sum1/1
  Product1/1 -> Normal Force/1, Product5/2
  Sum2/1 -> Saturation/1
  Saturation1/1 -> Product5/1  "mu*sign(v)"
  Demux3/1 -> Mux3/1
  Demux3/2 -> Mux3/2
  Selector3/1 -> Gain4/1
  Gain5/1 -> Sum5/1
  Gain4/1 -> Sum5/2
  Sum1/1 -> Demux3/1, Gain6/1
  Demux1/1 -> Mux1/1
  Demux1/2 -> Mux1/2
  Gain/1 -> Mux1/3
  Gain6/1 -> Demux1/1
  Constant1/1 -> Sum3/1
  Sum5/1 -> Sum4/1
  Selector2/1 -> Dot Product/1, Dot Product1/2
  Sum4/1 -> Gain1/1
  Mux3/1 -> FM/1
  Mux1/1 -> FM_rxn/1
  Saturation/1 -> Product1/1
  Dot Product1/1 -> Sum4/2

== system Drone_BBall_Developer/EMP Mechanics//Dynamics ==
  X_drone 1 : Inport
  X_drone 2 : Inport  Port=2
  fire_emp : Inport  Port=3
  AND : Logic  AllPortsSameDT=off  OutDataTypeStr=boolean
  AND1 : Logic  AllPortsSameDT=off  OutDataTypeStr=boolean
  Demux : Demux  Outputs=2
  Detect EMP Hit 1 : dspswit3/Edge Detector
      settings: SourceProductBaseCode=DS
  Detect EMP Hit 2 : dspswit3/Edge Detector
      settings: SourceProductBaseCode=DS
  Drone-EMP Collision 1 : Subsystem
  Drone-EMP Collision 2 : Subsystem
  Drone-EMP Logic 1 : Subsystem
  Drone-EMP Logic 2 : Subsystem
  EMP Dynamics 1 : Subsystem
  EMP Dynamics 2 : Subsystem
  Mux{1..4} (4 alike) : Mux  Inputs=2
  X_emp : Outport  VectorParamsAs1DForOutWhenUnconnected=off
  EMP Visible : Outport  Port=2  VectorParamsAs1DForOutWhenUnconnected=off
  EMP Armed : Outport  Port=3  VectorParamsAs1DForOutWhenUnconnected=off
  Stunned : Outport  Port=4  VectorParamsAs1DForOutWhenUnconnected=off
  wires:
  Drone-EMP Logic 1/4(EMP Live) -> AND/1
  Drone-EMP Logic 1/5(Reset EMP) -> EMP Dynamics 1/1(Reset)
  Drone-EMP Collision 1/1(Collision) -> AND/2
  Demux/2 -> Drone-EMP Logic 2/1(Fire EMP)
  EMP Dynamics 2/1("X_emp ") -> Mux3/2, Drone-EMP Collision 2/1(X_emp)
  Drone-EMP Logic 2/5(Reset EMP) -> EMP Dynamics 2/1(Reset)
  X_drone 2/1 -> Drone-EMP Collision 1/2(X_drone), EMP Dynamics 2/2(X_drone)
  Drone-EMP Logic 2/4(EMP Live) -> AND1/1
  Drone-EMP Collision 2/1(Collision) -> AND1/2
  AND/1 -> Detect EMP Hit 1/1
  AND1/1 -> Detect EMP Hit 2/1
  Detect EMP Hit 1/1 -> Drone-EMP Logic 2/3(Drone Hit), Drone-EMP Logic 1/2(EMP Hit)
  Detect EMP Hit 2/1 -> Drone-EMP Logic 2/2(EMP Hit), Drone-EMP Logic 1/3(Drone Hit)
  Drone-EMP Logic 1/2(EMP Visible) -> Mux1/1
  Mux1/1 -> EMP Visible/1
  Drone-EMP Logic 2/2(EMP Visible) -> Mux1/2
  Mux2/1 -> Stunned/1
  Drone-EMP Logic 1/1(Stunned) -> Mux2/1
  Drone-EMP Logic 2/1(Stunned) -> Mux2/2
  EMP Dynamics 1/1("X_emp ") -> Mux3/1, Drone-EMP Collision 1/1(X_emp)
  X_drone 1/1 -> EMP Dynamics 1/2(X_drone), Drone-EMP Collision 2/2(X_drone)
  Mux3/1 -> X_emp/1
  Drone-EMP Logic 1/3(EMP Armed) -> Mux4/1
  Drone-EMP Logic 2/3(EMP Armed) -> Mux4/2
  Mux4/1 -> EMP Armed/1
  fire_emp/1 -> Demux/1
  Demux/1 -> Drone-EMP Logic 1/1(Fire EMP)

== system Drone_BBall_Developer/Hoop Collision//Scoring ==
  X_ball : Inport
  F_drone_1 : Inport  Port=2
  F_drone_2 : Inport  Port=3
  Constant2 : Constant  Value=p_hoop(:,2)
  Constant4 : Constant  Value=p_hoop(:,3)
  Constant5 : Constant  Value=p_hoop(:,1)
  Constant7 : Constant  Value=p_hoop(:,4)
  Hoop Collision 1 : Subsystem
  Hoop Collision 2 : Subsystem
  Hoop Collision 3 : Subsystem
  Hoop Collision 4 : Subsystem
  Mux : Mux  Inputs=2
  NOT : Logic  Operator=NOT  IconShape=distinctive  AllPortsSameDT=off  OutDataTypeStr=boolean
  NOT1 : Logic  Operator=NOT  IconShape=distinctive  AllPortsSameDT=off  OutDataTypeStr=boolean
  OR : Logic  Operator=OR  AllPortsSameDT=off  OutDataTypeStr=boolean
  OR1 : Logic  AllPortsSameDT=off  OutDataTypeStr=boolean
  Score Detect 1 : Subsystem
  Score Detect 2 : Subsystem
  Sum4 : Sum  Inputs=++++
  Score : Outport  VectorParamsAs1DForOutWhenUnconnected=off
  Reset : Outport  Port=2  VectorParamsAs1DForOutWhenUnconnected=off
  FM_hoop : Outport  Port=3  VectorParamsAs1DForOutWhenUnconnected=off
  Live Ball : Outport  Port=4  VectorParamsAs1DForOutWhenUnconnected=off
  wires:
  X_ball/1 -> Hoop Collision 3/2(X_ball), Score Detect 2/3(X_ball), Hoop Collision 4/2(X_ball), Score Detect 1/3(X_ball), Hoop Collision 2/2(X_ball), Hoop Collision 1/2(X_ball)
  Hoop Collision 3/1(FM) -> Sum4/3
  Constant5/1 -> Score Detect 1/1(p_hoop L), Hoop Collision 1/1(p_hoop)
  Constant4/1 -> Score Detect 2/1(p_hoop L), Hoop Collision 3/1(p_hoop)
  Constant7/1 -> Score Detect 2/2(p_hoop R), Hoop Collision 4/1(p_hoop)
  Hoop Collision 2/1(FM) -> Sum4/2
  Hoop Collision 4/1(FM) -> Sum4/4
  Hoop Collision 1/1(FM) -> Sum4/1
  Sum4/1 -> FM_hoop/1
  Constant2/1 -> Score Detect 1/2(p_hoop R), Hoop Collision 2/1(p_hoop)
  Score Detect 1/2(Reset) -> OR/1
  Score Detect 2/2(Reset) -> OR/2
  OR/1 -> Reset/1
  Score Detect 2/1(Score) -> Mux/2
  Score Detect 1/1(Score) -> Mux/1
  Mux/1 -> Score/1
  Score Detect 1/3(Live) -> NOT/1, OR1/1
  Score Detect 2/3(Live) -> OR1/2, NOT1/1
  OR1/1 -> Live Ball/1
  NOT/1 -> Hoop Collision 2/3(in_net), Hoop Collision 1/3(in_net)
  NOT1/1 -> Hoop Collision 4/3(in_net), Hoop Collision 3/3(in_net)
  F_drone_1/1 -> Score Detect 1/4(F_ball)
  F_drone_2/1 -> Score Detect 2/4(F_ball)

== system Drone_BBall_Developer/Qualification Drone Controller ==
  X_drone : Inport
  X_ball : Inport  Port=2
  X_opponent : Inport  Port=3
  F_tether : Inport  Port=4
  EMP armed : Inport  Port=5
  Qualification Drone Controller_sfcn : S-Function  FunctionName=Qualification_sf  SFunctionModules=""  SFunctionDeploymentMode=off  EnableBusSupport=off  mask{rtw_sf_name=Qualification_sf, showVar=off}
      mask prompts: rtw_sf_name "Simulink:masks:GenSFuncName_MP"; showVar "Simulink:masks:GenSFuncShowModuleList_MP"
      mask help: Simulink:masks:GenSFuncDesc_MD
      mask init:
      | displist = '';
      | if ~strcmp(get_param(gcb, 'FunctionName'), rtw_sf_name);
      |   set_param(gcb, 'FunctionName', rtw_sf_name);
      | end
      | % Check if we are generating code
      | rtw_mode = false;
      | if strcmpi(get_param(bdroot(gcb),'SimulationStatus'),'Initializing')
      | 	rtw_mode = strcmpi(get_param(bdroot(gcb),'BuildingRTWCode'),'on') && ...
      | 		~strcmpi(get_param(bdroot(gcb),'TargetStyle'),'SimulationTarget');
      | end
      | if showVar || rtw_mode
      | 	if exist('rtwsfunc') == 2 | exist('rtwsfunc') == 6
      | 		tmplist = rtwsfunc(rtw_sf_name,gcb);
      | 		tmplist = DAStudio.message('Simulink:masks:GenSFuncListOfModules_IC', tmplist);
      | 	elseif showVar
      | 		tmplist1 = DAStudio.message('Simulink:masks:GenSFuncListOfModules_IC', '');
      |         tmplist2 = DAStudio.message('Simulink:masks:GenSFuncNotLicensed_IC');
      |         tmplist = [tmplist1 tmplist2];
      |  	end
      | end
      | if showVar
      |   displist = tmplist;
      | end
      settings: CopyFcn=|
      | if ~strcmp(get_param(gcb,'Linkstatus'),'none') && ...
      | ~strcmp(get_param(gcb,'Linkstatus'),'implicit')
      |   set_param(gcb,'LinkStatus','none');
      | end
      mask Help: eval('feval(''rtwprivate'',''rtwhelpview'',''rtw_sfcn_block'')');
      mask Display:
      | port_label('input',1,'X_drone');
      | port_label('input',2,'X_ball');
      | port_label('input',3,'X_opponent');
      | port_label('input',4,'F_tether');
      | port_label('input',5,'EMP armed');
      | port_label('output',1,'fire_emp');
      | port_label('output',2,'mag_on');
      | port_label('output',3,'T_L_d');
      | port_label('output',4,'T_R_d');
      | port_label('output',5,'X_d');
  __InputSSForSFun__ : Subsystem
  __OutputSSForSFun__ : Subsystem
  fire_emp : Outport  VectorParamsAs1DForOutWhenUnconnected=off
  mag_on : Outport  Port=2  VectorParamsAs1DForOutWhenUnconnected=off
  T_L_d : Outport  Port=3  VectorParamsAs1DForOutWhenUnconnected=off
  T_R_d : Outport  Port=4  VectorParamsAs1DForOutWhenUnconnected=off
  X_d : Outport  Port=5  VectorParamsAs1DForOutWhenUnconnected=off
  wires:
  X_drone/1 -> __InputSSForSFun__/1(X_drone)
  X_ball/1 -> __InputSSForSFun__/2(X_ball)
  X_opponent/1 -> __InputSSForSFun__/3(X_opponent)
  F_tether/1 -> __InputSSForSFun__/4(F_tether)
  EMP armed/1 -> __InputSSForSFun__/5(EMP armed)
  __InputSSForSFun__/1(__UniqueOutportName__1__) -> Qualification Drone Controller_sfcn/1
  __InputSSForSFun__/2(__UniqueOutportName__2__) -> Qualification Drone Controller_sfcn/2
  __InputSSForSFun__/3(__UniqueOutportName__3__) -> Qualification Drone Controller_sfcn/3
  __InputSSForSFun__/4(__UniqueOutportName__4__) -> Qualification Drone Controller_sfcn/4
  __InputSSForSFun__/5(__UniqueOutportName__5__) -> Qualification Drone Controller_sfcn/5
  Qualification Drone Controller_sfcn/1 -> __OutputSSForSFun__/1(__UniqueInportName__1__)
  Qualification Drone Controller_sfcn/2 -> __OutputSSForSFun__/2(__UniqueInportName__2__)
  Qualification Drone Controller_sfcn/3 -> __OutputSSForSFun__/3(__UniqueInportName__3__)
  Qualification Drone Controller_sfcn/4 -> __OutputSSForSFun__/4(__UniqueInportName__4__)
  Qualification Drone Controller_sfcn/5 -> __OutputSSForSFun__/5(__UniqueInportName__5__)
  __OutputSSForSFun__/1(fire_emp) -> fire_emp/1
  __OutputSSForSFun__/2(mag_on) -> mag_on/1
  __OutputSSForSFun__/3(T_L_d) -> T_L_d/1
  __OutputSSForSFun__/4(T_R_d) -> T_R_d/1
  __OutputSSForSFun__/5(X_d) -> X_d/1

== system Drone_BBall_Developer/Ball Dynamics/Ceiling Reactions ==
  X : Inport
  Constant : Constant  Value=0
  Constant1 : Constant  Value=16-r_ball
  Demux : Demux  Outputs=6
  Gain : Gain  Gain=-k_F_R_ball
  Gain1 : Gain  Gain=r_ball
  Gain2 : Gain  Gain=r_ball
  Gain3 : Gain  Gain=-k_f
  Gain4 : Gain  Gain=-b_F_R_ball
  Less Than : RelationalOperator  Operator=<  OutDataTypeStr=boolean  RndMeth=Simplest
  Mux : Mux  Inputs=3
  Product1 : Product
  Product4 : Product  Inputs=3
  Saturation : Saturate  UpperLimit=0  LowerLimit=-Inf
  Saturation1 : Saturate  UpperLimit=mu_f  LowerLimit=-mu_f
  Sum : Sum  Inputs=|++
  Sum1 : Sum  Inputs=-+|
  Sum2 : Sum  Inputs=--|
  Terminator : Terminator
  Terminator1 : Terminator
  FM_R : Outport  VectorParamsAs1DForOutWhenUnconnected=off
  wires:
  Demux/4 -> Gain4/1
  Constant/1 -> Less Than/1
  Sum/1 -> Saturation/1
  Gain4/1 -> Sum/2
  Gain/1 -> Sum/1
  Sum2/1 -> Gain3/1
  Demux/2 -> Sum2/1
  Less Than/1 -> Product4/3, Product1/1
  Product4/1 -> Mux/1, Gain1/1
  Demux/3 -> Sum1/2
  Constant1/1 -> Sum1/1
  Sum1/1 -> Less Than/2, Gain/1
  Demux/6 -> Gain2/1
  Product1/1 -> Mux/2
  Mux/1 -> FM_R/1
  Demux/1 -> Terminator/1
  Demux/5 -> Terminator1/1
  X/1 -> Demux/1
  Saturation/1 -> Product1/2, Product4/2
  Saturation1/1 -> Product4/1
  Gain3/1 -> Saturation1/1
  Gain2/1 -> Sum2/2
  Gain1/1 -> Mux/3

== system Drone_BBall_Developer/Ball Dynamics/Ground Reactions ==
  X : Inport
  Constant : Constant  Value=0
  Constant1 : Constant  Value=r_ball
  Demux : Demux  Outputs=6
  Gain : Gain  Gain=-k_F_R_ball
  Gain1 : Gain  Gain=-r_ball
  Gain2 : Gain  Gain=r_ball
  Gain3 : Gain  Gain=-k_f
  Gain4 : Gain  Gain=-b_F_R_ball
  Less Than : RelationalOperator  Operator=>  OutDataTypeStr=boolean  RndMeth=Simplest
  Mux : Mux  Inputs=3
  Product1 : Product
  Product4 : Product  Inputs=3
  Saturation : Saturate  UpperLimit=Inf  LowerLimit=0
  Saturation1 : Saturate  UpperLimit=mu_f  LowerLimit=-mu_f
  Sum : Sum  Inputs=|++
  Sum1 : Sum  Inputs=-+|
  Sum2 : Sum  Inputs=+-|
  Terminator : Terminator
  Terminator1 : Terminator
  FM_R : Outport  VectorParamsAs1DForOutWhenUnconnected=off
  wires:
  Demux/4 -> Gain4/1
  Constant/1 -> Less Than/1
  Sum/1 -> Saturation/1
  Gain4/1 -> Sum/2
  Gain/1 -> Sum/1
  Sum2/1 -> Gain3/1
  Demux/2 -> Sum2/1
  Less Than/1 -> Product4/3, Product1/1
  Product4/1 -> Mux/1, Gain1/1
  Demux/3 -> Sum1/2
  Constant1/1 -> Sum1/1
  Sum1/1 -> Less Than/2, Gain/1
  Demux/6 -> Gain2/1
  Product1/1 -> Mux/2
  Mux/1 -> FM_R/1
  Demux/1 -> Terminator/1
  Demux/5 -> Terminator1/1
  X/1 -> Demux/1
  Saturation/1 -> Product1/2, Product4/2
  Saturation1/1 -> Product4/1
  Gain3/1 -> Saturation1/1
  Gain2/1 -> Sum2/2
  Gain1/1 -> Mux/3

== system Drone_BBall_Developer/Ball Dynamics/Left Wall Reactions ==
  X : Inport
  Constant : Constant  Value=0
  Constant1 : Constant  Value=-12+r_ball
  Demux : Demux  Outputs=6
  Gain : Gain  Gain=-k_F_R_ball
  Gain1 : Gain  Gain=r_ball
  Gain2 : Gain  Gain=r_ball
  Gain3 : Gain  Gain=-k_f
  Gain4 : Gain  Gain=-b_F_R_ball
  Less Than : RelationalOperator  Operator=<  OutDataTypeStr=boolean  RndMeth=Simplest
  Mux : Mux  Inputs=3
  Product1 : Product
  Product4 : Product  Inputs=3
  Saturation : Saturate  UpperLimit=Inf  LowerLimit=0
  Saturation1 : Saturate  UpperLimit=mu_f  LowerLimit=-mu_f
  Sum : Sum  Inputs=|++
  Sum1 : Sum  Inputs=-+|
  Sum2 : Sum  Inputs=++|
  Terminator1 : Terminator
  Terminator2 : Terminator
  FM_R : Outport  VectorParamsAs1DForOutWhenUnconnected=off
  wires:
  Demux/2 -> Gain4/1
  Constant/1 -> Less Than/2
  Sum/1 -> Saturation/1
  Gain4/1 -> Sum/2
  Gain/1 -> Sum/1
  Sum2/1 -> Gain3/1
  Demux/4 -> Sum2/1
  Less Than/1 -> Product1/2, Product4/3
  Product4/1 -> Mux/2, Gain1/1
  Demux/1 -> Sum1/2
  Constant1/1 -> Sum1/1
  Sum1/1 -> Less Than/1, Gain/1
  Demux/6 -> Gain2/1
  Product1/1 -> Mux/1
  Mux/1 -> FM_R/1
  Demux/5 -> Terminator1/1
  X/1 -> Demux/1
  Saturation/1 -> Product4/2, Product1/1
  Saturation1/1 -> Product4/1
  Gain3/1 -> Saturation1/1
  Gain2/1 -> Sum2/2
  Gain1/1 -> Mux/3
  Demux/3 -> Terminator2/1

== system Drone_BBall_Developer/Ball Dynamics/Linear Dynamics ==
  Reset : Inport
  F : Inport  Port=2
  Band-Limited White Noise : simulink/Sources/Band-Limited White Noise  Cov=[.7^2]  Ts=0.1  seed=round(sum(clock))
  Constant : Constant  Value=p_ball_dot_0
  Constant1 : Constant  Value=0
  Gain1 : Gain  Gain=1/m_ball
  Gain4 : Gain  Gain=b_ball
  Integrator : Integrator  ExternalReset=rising  InitialConditionSource=external  InitialCondition=p_ball_dot_0
  Integrator1 : Integrator  ExternalReset=rising  InitialCondition=p_ball_0
  Mux : Mux  Inputs=2
  Norm : Fcn  Expr=sqrt(u(1)^2+u(2)^2)
  Product : Product
  Sum : Sum  Inputs=++|
  Sum2 : Sum  Inputs=+-
  p : Outport  VectorParamsAs1DForOutWhenUnconnected=off
  p_dot : Outport  Port=2  VectorParamsAs1DForOutWhenUnconnected=off
  wires:
  Sum2/1 -> Gain1/1
  Gain1/1 -> Integrator/1
  Product/1 -> Gain4/1
  F/1 -> Sum2/1
  Gain4/1 -> Sum2/2
  Norm/1 -> Product/2
  Reset/1 -> Integrator1/2, Integrator/2
  Integrator/1 -> Norm/1, p_dot/1, Product/1, Integrator1/1
  Integrator1/1 -> p/1
  Constant/1 -> Sum/1
  Sum/1 -> Integrator/3
  Constant1/1 -> Mux/1
  Band-Limited White Noise/1 -> Mux/2
  Mux/1 -> Sum/2

== system Drone_BBall_Developer/Ball Dynamics/Right Wall Reactions ==
  X : Inport
  Constant : Constant  Value=0
  Constant1 : Constant  Value=12-r_ball
  Demux : Demux  Outputs=6
  Gain : Gain  Gain=-k_F_R_ball
  Gain1 : Gain  Gain=-r_ball
  Gain2 : Gain  Gain=r_ball
  Gain3 : Gain  Gain=-k_f
  Gain4 : Gain  Gain=-b_F_R_ball
  Less Than : RelationalOperator  Operator=>  OutDataTypeStr=boolean  RndMeth=Simplest
  Mux : Mux  Inputs=3
  Product1 : Product
  Product4 : Product  Inputs=3
  Saturation : Saturate  UpperLimit=0  LowerLimit=-Inf
  Saturation1 : Saturate  UpperLimit=mu_f  LowerLimit=-mu_f
  Sum : Sum  Inputs=|++
  Sum1 : Sum  Inputs=-+|
  Sum2 : Sum  Inputs=-+|
  Terminator1 : Terminator
  Terminator2 : Terminator
  FM_R : Outport  VectorParamsAs1DForOutWhenUnconnected=off
  wires:
  Demux/2 -> Gain4/1
  Constant/1 -> Less Than/2
  Sum/1 -> Saturation/1
  Gain4/1 -> Sum/2
  Gain/1 -> Sum/1
  Sum2/1 -> Gain3/1
  Demux/4 -> Sum2/1
  Less Than/1 -> Product1/2, Product4/3
  Product4/1 -> Mux/2, Gain1/1
  Demux/1 -> Sum1/2
  Constant1/1 -> Sum1/1
  Sum1/1 -> Less Than/1, Gain/1
  Demux/6 -> Gain2/1
  Product1/1 -> Mux/1
  Mux/1 -> FM_R/1
  Demux/5 -> Terminator1/1
  X/1 -> Demux/1
  Saturation/1 -> Product4/2, Product1/1
  Saturation1/1 -> Product4/1
  Gain3/1 -> Saturation1/1
  Gain2/1 -> Sum2/2
  Gain1/1 -> Mux/3
  Demux/3 -> Terminator2/1

== system Drone_BBall_Developer/Ball Dynamics/Rotational Dynamics ==
  Reset : Inport
  M : Inport  Port=2
  Fcn : Fcn  Expr=u*abs(u)
  Gain : Gain  Gain=b_th_ball
  Gain1 : Gain  Gain=1/J_ball
  Integrator : Integrator  ExternalReset=rising
  Integrator1 : Integrator  ExternalReset=rising
  Sum2 : Sum  Inputs=|+-
  Wrap Angle : Subsystem
  theta : Outport  VectorParamsAs1DForOutWhenUnconnected=off
  theta_dot : Outport  Port=2  VectorParamsAs1DForOutWhenUnconnected=off
  wires:
  Integrator1/1 -> Wrap Angle/1(raw)
  Integrator/1 -> Integrator1/1, theta_dot/1, Fcn/1
  Sum2/1 -> Gain1/1
  Gain1/1 -> Integrator/1
  M/1 -> Sum2/1
  Gain/1 -> Sum2/2
  Wrap Angle/1(wrap) -> theta/1
  Fcn/1 -> Gain/1
  Reset/1 -> Integrator1/2, Integrator/2

== system Drone_BBall_Developer/Drone 1 Controller/Detect Ball in Freefall ==
  X : Inport
  AND : Logic  AllPortsSameDT=off  OutDataTypeStr=boolean
  Constant : Constant  Value=-g+g_tol
  Constant1 : Constant  Value=-g-g_tol
  Derivative : Derivative
  GreaterThan : RelationalOperator  Operator=>  OutDataTypeStr=boolean  RndMeth=Simplest
  GreaterThan1 : RelationalOperator  Operator=>  OutDataTypeStr=boolean  RndMeth=Simplest
  Scope2 : Scope
  Selector : Selector  InputPortWidth=6  IndexOptions=Index vector (dialog)  Indices=[4]  OutputSizes=1
  Object in Freefall : Outport
  wires:
  X/1 -> Selector/1
  Selector/1 -> Derivative/1
  Derivative/1 -> GreaterThan/1, Scope2/1, GreaterThan1/2
  GreaterThan1/1 -> AND/1
  GreaterThan/1 -> AND/2
  Constant/1 -> GreaterThan1/1
  Constant1/1 -> GreaterThan/2
  AND/1 -> Object in Freefall/1

== system Drone_BBall_Developer/Drone 1 Controller/Preamp to smooth p_d(t) (Double click to tune) ==
  X_d_raw(t) : Inport
  Demux : Demux  Outputs=6
  Derivative : Derivative  CoefficientInTFapproximation=.01
  Derivative1 : Derivative  CoefficientInTFapproximation=.01
  Derivative2 : Derivative  CoefficientInTFapproximation=.01
  Gain : Gain  Gain=pi/180
  Mux : Mux  Inputs=6
  Reference Trajectory Filters : simulink_extras/Additional Linear/Transfer Fcn (with initial states)  N=[omega_th^2]  D=[1 2*zeta_th*omega_th omega_th^2]  X0=[0; 0]/omega_th^2
  Scope : Scope  NumInputPorts=2
  Terminator : Terminator
  Terminator1 : Terminator
  Terminator2 : Terminator
  Transfer Fcn : simulink_extras/Additional Linear/Transfer Fcn (with initial states)  N=[omega_y^2]  D=[1 2*zeta_y*omega_y omega_y^2]  X0=[0; p_0(2)]/omega_y^2
  Transfer Fcn (with initial states) : simulink_extras/Additional Linear/Transfer Fcn (with initial states)  N=[omega_x^2]  D=[1 2*zeta_x*omega_x omega_x^2]  X0=[0; p_0(1)]/omega_x^2
  X_d(t) : Outport  VectorParamsAs1DForOutWhenUnconnected=off
  wires:
  Demux/3 -> Transfer Fcn/1
  Transfer Fcn (with initial states)/1 -> Derivative/1, Mux/1
  Transfer Fcn/1 -> Derivative1/1, Mux/3
  X_d_raw(t)/1 -> Scope/1, Demux/1  "X_d_raw"
  Demux/1 -> Transfer Fcn (with initial states)/1
  Mux/1 -> Scope/2, X_d(t)/1  "X_d"
  Derivative/1 -> Mux/2
  Derivative1/1 -> Mux/4
  Derivative2/1 -> Mux/6
  Demux/5 -> Gain/1
  Gain/1 -> Reference Trajectory Filters/1
  Reference Trajectory Filters/1 -> Derivative2/1, Mux/5
  Demux/2 -> Terminator/1
  Demux/4 -> Terminator1/1
  Demux/6 -> Terminator2/1
